simulink model "algorithm"  (R2026a)
settings: Solver=FixedStepDiscrete  FixedStep=foc.Ts
PreLoadFcn:
  | if exist('init', 'file') ~= 2,   pDir = fileparts(fileparts(which(bdroot)));   if isempty(pDir), pDir = pwd; end;   addpath(fullfile(pDir, 'scripts'));   addpath(fullfile(pDir, 'models'));   addpath(pDir); end; init;
InitFcn:
  | if exist('init', 'file') ~= 2,   pDir = fileparts(fileparts(which(bdroot)));   if isempty(pDir), pDir = pwd; end;   addpath(fullfile(pDir, 'scripts'));   addpath(fullfile(pDir, 'models'));   addpath(pDir); end; init;
undefined symbols (not defined in the file): calibration_modulation, calibration_request, control_enable_request, control_fault_reset, control_mode_request, current_offset_counts, DiscIntNeverNeededParam, foc, has_stored_resolver_offset, open_loop_electrical_hz, open_loop_modulation, pmsm, resolver_angle_offset, sensor, torque_ref_nm
libraries: mcbeeMathTransformLib x3, slpidlib x3, mcbcontrolslib x3, simulink x2, mcbpositiondecoderlib x1
(part 2 of 2)

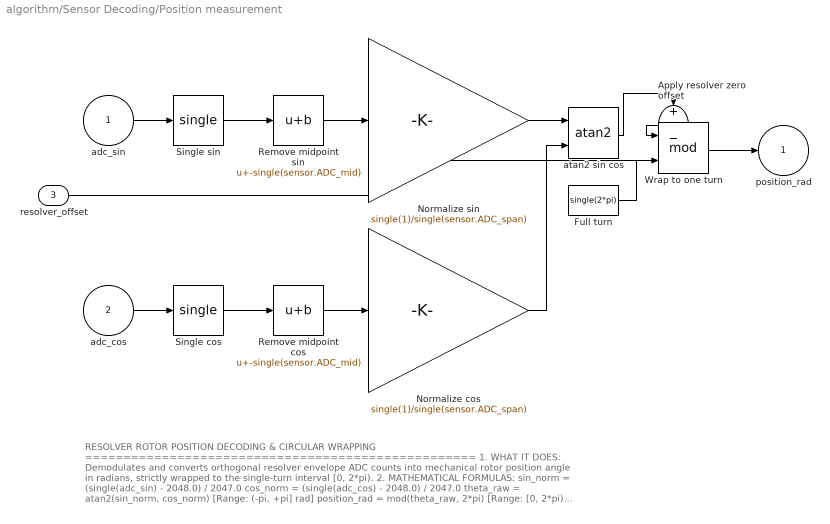
== system algorithm/Sensor Decoding/Position measurement ==
  note: RESOLVER ROTOR POSITION DECODING & CIRCULAR WRAPPING
      | ===================================================
      | 1. WHAT IT DOES:
      | Demodulates and converts orthogonal resolver envelope ADC counts into mechanical rotor
      | position angle in radians, strictly wrapped to the single-turn interval [0, 2*pi).
      |
      | 2. MATHEMATICAL FORMULAS:
      |   sin_norm = (single(adc_sin) - 2048.0) / 2047.0
      |   cos_norm = (single(adc_cos) - 2048.0) / 2047.0
      |   theta_raw = atan2(sin_norm, cos_norm)           [Range: (-pi, +pi] rad]
      |   position_rad = mod(theta_raw, 2*pi)             [Range: [0, 2*pi) rad]
      |
      | 3. WHY IT IS NEEDED:
      | Field-Oriented Control requires accurate, continuous knowledge of rotor position to align
      | the Park and Clarke reference frames. Using atan2(sin, cos) provides amplitude-invariant
      | angle reconstruction that rejects common-mode excitation variations and noise. Wrapping to
      | [0, 2*pi) provides a clean, standardized mechanical coordinate system for electrical angle derivation.
  adc_sin : Inport  OutDataTypeStr=uint16
  adc_cos : Inport  Port=2  OutDataTypeStr=uint16
  resolver_offset : Inport  Port=3
  Apply resolver zero offset : Sum  Inputs=+-
  Full turn : Constant  Value=single(2*pi)
  Normalize cos : Gain  Gain=single(1)/single(sensor.ADC_span)
  Normalize sin : Gain  Gain=single(1)/single(sensor.ADC_span)
  Remove midpoint cos : Bias  Bias=-single(sensor.ADC_mid)
  Remove midpoint sin : Bias  Bias=-single(sensor.ADC_mid)
  Single cos : DataTypeConversion  OutDataTypeStr=single
  Single sin : DataTypeConversion  OutDataTypeStr=single
  Wrap to one turn : Math  Operator=mod
  atan2 sin cos : Trigonometry  Operator=atan2
  position_rad : Outport
  wires:
  Wrap to one turn/1 -> position_rad/1
  Normalize cos/1 -> atan2 sin cos/2
  Normalize sin/1 -> atan2 sin cos/1
  Remove midpoint cos/1 -> Normalize cos/1
  adc_cos/1 -> Single cos/1
  Remove midpoint sin/1 -> Normalize sin/1
  Single cos/1 -> Remove midpoint cos/1
  Single sin/1 -> Remove midpoint sin/1
  Full turn/1 -> Wrap to one turn/2
  adc_sin/1 -> Single sin/1
  atan2 sin cos/1 -> Apply resolver zero offset/1
  Apply resolver zero offset/1 -> Wrap to one turn/1
  resolver_offset/1 -> Apply resolver zero offset/2

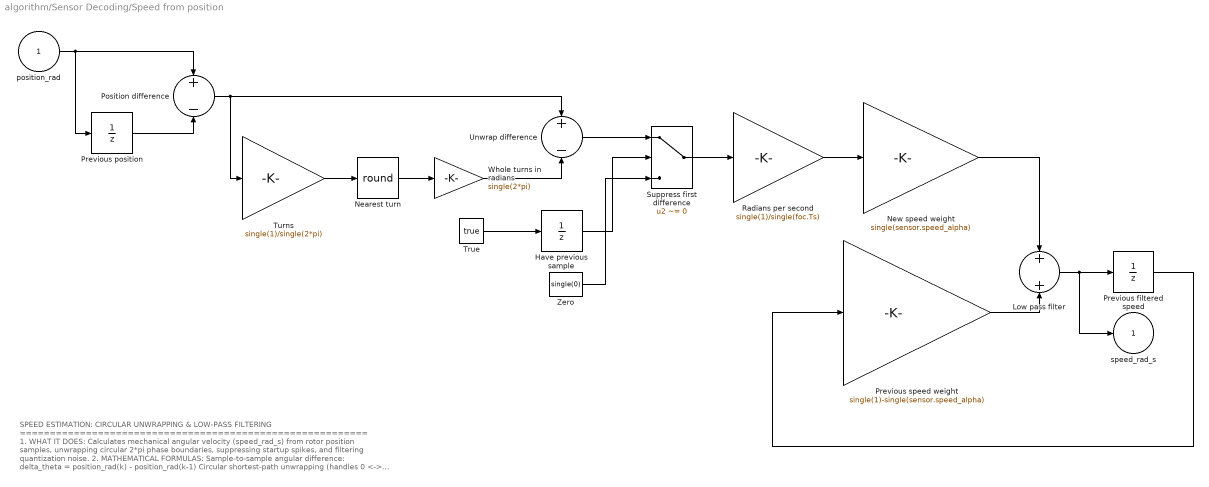
== system algorithm/Sensor Decoding/Speed from position ==
  note: SPEED ESTIMATION: CIRCULAR UNWRAPPING & LOW-PASS FILTERING
      | ==========================================================
      | 1. WHAT IT DOES:
      | Calculates mechanical angular velocity (speed_rad_s) from rotor position samples,
      | unwrapping circular 2*pi phase boundaries, suppressing startup spikes, and filtering
      | quantization noise.
      |
      | 2. MATHEMATICAL FORMULAS:
      | Sample-to-sample angular difference:
      |   delta_theta = position_rad(k) - position_rad(k-1)
      |
      | Circular shortest-path unwrapping (handles 0 <-> 2*pi transitions):
      |   delta_theta_unwrap = delta_theta - 2*pi * round(delta_theta / (2*pi))
      |
      | Differentiated raw speed (with first-step startup suppression):
      |   omega_raw(1) = 0
      |   omega_raw(k) = delta_theta_unwrap / Ts          [Ts = 50 us (20 kHz)]
      |
      | Discrete 1st-order Low-Pass Filter (cutoff fc = 150 Hz):
      |   omega_filt(k) = (1 - alpha) * omega_filt(k-1) + alpha * omega_raw(k)
      |   alpha = (2*pi * fc * Ts) / (1 + 2*pi * fc * Ts) ≈ 0.04505
      |
      | 3. WHY IT IS NEEDED:
      | - Boundary Wrap Immunity: As the rotor rotates past 2*pi -> 0 or 0 -> 2*pi, delta_theta
      |   would jump by +/-2*pi, producing an enormous false velocity spike (+/-125,663 rad/s).
      |   Shortest-path unwrapping eliminates this completely.
      | - Startup Quiescence: Suppressing the first step prevents false speed kicks when starting
      |   from a nonzero stationary angle.
      | - Noise Rejection: Differentiating quantized 12-bit ADC resolver signals amplifies high-
      |   frequency quantization noise; the 150 Hz LPF smooths the velocity signal for stable speed
      |   and current loop feedback.
  position_rad : Inport  OutDataTypeStr=single
  Have previous sample : UnitDelay  InitialCondition=false  SampleTime=foc.Ts
  Low pass filter : Sum
  Nearest turn : Rounding  Operator=round
  New speed weight : Gain  Gain=single(sensor.speed_alpha)
  Position difference : Sum  Inputs=+-
  Previous filtered speed : UnitDelay  InitialCondition=single(0)  SampleTime=foc.Ts
  Previous position : UnitDelay  InitialCondition=single(0)  SampleTime=foc.Ts
  Previous speed weight : Gain  Gain=single(1)-single(sensor.speed_alpha)
  Radians per second : Gain  Gain=single(1)/single(foc.Ts)
  Suppress first difference : Switch  Criteria=u2 ~= 0
  True : Constant  Value=true
  Turns : Gain  Gain=single(1)/single(2*pi)
  Unwrap difference : Sum  Inputs=+-
  Whole turns in radians : Gain  Gain=single(2*pi)
  Zero : Constant  Value=single(0)
  speed_rad_s : Outport
  wires:
  Previous filtered speed/1 -> Previous speed weight/1
  Previous speed weight/1 -> Low pass filter/2
  New speed weight/1 -> Low pass filter/1
  Radians per second/1 -> New speed weight/1
  Unwrap difference/1 -> Suppress first difference/1
  Position difference/1 -> Turns/1, Unwrap difference/1
  Nearest turn/1 -> Whole turns in radians/1
  Suppress first difference/1 -> Radians per second/1
  position_rad/1 -> Previous position/1, Position difference/1
  Turns/1 -> Nearest turn/1
  Low pass filter/1 -> speed_rad_s/1, Previous filtered speed/1
  Have previous sample/1 -> Suppress first difference/2
  Zero/1 -> Suppress first difference/3
  Whole turns in radians/1 -> Unwrap difference/2
  Previous position/1 -> Position difference/2
  True/1 -> Have previous sample/1

== matlab function algorithm/Sensor Offset Calibration/Average and store offsets ==
  data: ia input size=1; current_offsets output size=[3]; ib input size=1; ic input size=1; rsin input size=1; rcos input size=1; current_enable input size=1; resolver_enable input size=1; current_initial input size=[3]; resolver_initial input size=1; resolver_offset output size=1; current_done output size=1; resolver_done output size=1
function [current_offsets, resolver_offset, current_done, resolver_done] = calibrate(ia, ib, ic, rsin, rcos, current_enable, resolver_enable, current_initial, resolver_initial)
%#codegen
% Signal averaging belongs in Simulink. Stateflow only enables each phase.
persistent current_store resolver_store current_sum resolver_sin_sum resolver_cos_sum current_count resolver_count previous_current_enable previous_resolver_enable
if isempty(current_store)
    current_store = single(current_initial);
    resolver_store = single(resolver_initial);
    current_sum = single([0;0;0]);
    resolver_sin_sum = single(0); resolver_cos_sum = single(0);
    current_count = uint32(0); resolver_count = uint32(0);
    previous_current_enable = false; previous_resolver_enable = false;
end
current_done = false; resolver_done = false;
if current_enable
    if ~previous_current_enable
        current_sum = single([0;0;0]); current_count = uint32(0);
    end
    if current_count < uint32(10000)
        current_sum = current_sum + single([ia;ib;ic]);
        current_count = current_count + uint32(1);
    end
    if current_count >= uint32(10000)
        current_store = current_sum / single(current_count); current_done = true;
    end
end
if resolver_enable
    if ~previous_resolver_enable
        resolver_sin_sum = single(0); resolver_cos_sum = single(0); resolver_count = uint32(0);
    end
    if resolver_count < uint32(10000)
        resolver_sin_sum = resolver_sin_sum + single(rsin) - single(2048);
        resolver_cos_sum = resolver_cos_sum + single(rcos) - single(2048);
        resolver_count = resolver_count + uint32(1);
    end
    if resolver_count >= uint32(10000)
        resolver_store = atan2(resolver_sin_sum, resolver_cos_sum); resolver_done = true;
    end
end
previous_current_enable = current_enable;
previous_resolver_enable = resolver_enable;
current_offsets = current_store;
resolver_offset = resolver_store;
end

== matlab function algorithm/Protection Monitor ==
  data: currents input single size=[3]; fault output boolean size=1; speed input single size=1; ia input uint16 size=1; ib input uint16 size=1; ic input uint16 size=1; rsin input uint16 size=1; rcos input uint16 size=1; reset input; fault_flags output
function [fault, fault_flags] = protection_monitor(currents, speed, ia, ib, ic, rsin, rcos, reset)
%#codegen
rawCurrent = abs(single(currents));
oc_u = rawCurrent(1) > single(0.90);
oc_v = rawCurrent(2) > single(0.90);
oc_w = rawCurrent(3) > single(0.90);
overcurrent = oc_u || oc_v || oc_w;

overspeed = abs(speed) > single(2094.3951);

rail_low  = (ia <= uint16(8)) || (ib <= uint16(8)) || (ic <= uint16(8));
rail_high = (ia >= uint16(4087)) || (ib >= uint16(4087)) || (ic >= uint16(4087));
adcRail   = rail_low || rail_high;

s = (single(rsin) - single(2048)) / single(2047);
c = (single(rcos) - single(2048)) / single(2047);
amp = sqrt(s*s + c*c);
res_low  = amp < single(0.10);
res_high = amp > single(1.30);
resolverBad = res_low || res_high;

persistent bad_count latched_flags
if isempty(bad_count)
    bad_count = uint16(0);
    latched_flags = uint32(0);
end

bad = overcurrent || overspeed || adcRail || resolverBad;
if bad
    if bad_count < uint16(100)
        bad_count = bad_count + uint16(1);
    end
else
    bad_count = uint16(0);
end

fault = (bad_count >= uint16(100));

% Active fault bits:
active_flags = uint32(0);
if oc_u,      active_flags = bitor(active_flags, uint32(1)); end    % Bit 0: Overcurrent U
if oc_v,      active_flags = bitor(active_flags, uint32(2)); end    % Bit 1: Overcurrent V
if oc_w,      active_flags = bitor(active_flags, uint32(4)); end    % Bit 2: Overcurrent W
if overspeed, active_flags = bitor(active_flags, uint32(8)); end    % Bit 3: Overspeed
if rail_low,  active_flags = bitor(active_flags, uint32(16)); end   % Bit 4: ADC Rail Low
if rail_high, active_flags = bitor(active_flags, uint32(32)); end   % Bit 5: ADC Rail High
if res_low,   active_flags = bitor(active_flags, uint32(64)); end   % Bit 6: Resolver Amp Low
if res_high,  active_flags = bitor(active_flags, uint32(128)); end  % Bit 7: Resolver Amp High
if fault,     active_flags = bitor(active_flags, uint32(256)); end  % Bit 8: Trip Latched

if reset
    latched_flags = active_flags;
else
    latched_flags = bitor(latched_flags, active_flags);
end

fault_flags = latched_flags;
end

== stateflow chart algorithm/Operating Mode Supervisor ==
  state IDLE
    entry:
    supervisor_state = SupervisorState.IDLE;
    active_mode = uint8(0);
    pwm_enable = false;
    current_cal_enable = false;
    resolver_align_enable = false;
    resolver_sample_enable = false;
    fault_latched = false;
    during:
    if calibration_request == uint8(0)
    cal_request_processed = false;
    end
  state READY
    entry:
    supervisor_state = SupervisorState.READY;
    active_mode = uint8(0);
    pwm_enable = false;
    current_cal_enable = false;
    resolver_align_enable = false;
    resolver_sample_enable = false;
    fault_latched = false;
    during:
    if ~enable_request
    reenable_required = false;
    end
    if calibration_request == uint8(0)
    cal_request_processed = false;
    end
  state RUN
    entry:
    supervisor_state = SupervisorState.RUN;
    run_mode = mode_request;
    active_mode = run_mode;
    pwm_enable = true;
    current_cal_enable = false;
    resolver_align_enable = false;
    resolver_sample_enable = false;
    fault_latched = false;
    during:
    active_mode = run_mode;
    if calibration_request == uint8(0)
    cal_request_processed = false;
    end
  state CALIBRATION
    entry:
    supervisor_state = SupervisorState.CALIBRATION;
    active_mode = uint8(0);
    pwm_enable = false;
    current_cal_enable = false;
    resolver_align_enable = false;
    resolver_sample_enable = false;
    do_current_cal = ~startup_current_cal_done || calibration_request == uint8(1) || calibration_request == uint8(3);
    do_angle_cal = ~has_stored_angle || calibration_request == uint8(2) || calibration_request == uint8(3);
    fault_latched = false;
    state CURRENT_CAL
      entry:
      current_cal_enable = true;
      pwm_enable = false;
      resolver_align_enable = false;
      resolver_sample_enable = false;
      exit:
      current_cal_enable = false;
      startup_current_cal_done = true;
    state ANGLE_ALIGN
      entry:
      current_cal_enable = false;
      pwm_enable = true;
      resolver_align_enable = true;
      resolver_sample_enable = false;
      ticks = uint32(0);
      during:
      ticks = ticks + uint32(1);
    state ANGLE_SAMPLE
      entry:
      current_cal_enable = false;
      pwm_enable = true;
      resolver_align_enable = true;
      resolver_sample_enable = true;
    state CAL_DONE
      entry:
      current_cal_enable = false;
      pwm_enable = false;
      resolver_align_enable = false;
      resolver_sample_enable = false;
      cal_request_processed = true;
    state SELECT_CALIBRATION
      entry:
      pwm_enable = false;
    CURRENT_CAL -> ANGLE_ALIGN [order 1] : [current_cal_done && do_angle_cal]
    ANGLE_ALIGN -> ANGLE_SAMPLE : [ticks >= uint32(20000)]
    ANGLE_SAMPLE -> CAL_DONE : [resolver_cal_done]
    SELECT_CALIBRATION -> CURRENT_CAL [order 1] : [do_current_cal]
    CURRENT_CAL -> CAL_DONE [order 2] : [current_cal_done && ~do_angle_cal]
    SELECT_CALIBRATION -> ANGLE_ALIGN [order 2] : [~do_current_cal && do_angle_cal]
    SELECT_CALIBRATION -> CAL_DONE [order 3]
  state FAULT
    entry:
    supervisor_state = SupervisorState.FAULT;
    active_mode = uint8(0);
    pwm_enable = false;
    current_cal_enable = false;
    resolver_align_enable = false;
    resolver_sample_enable = false;
    fault_latched = true;
  RUN -> IDLE [order 2] : [mode_request == uint8(0) || mode_request > uint8(3)]
  (default) -> SELECT_CALIBRATION [order 1]
  (default) -> IDLE [order 2]
  IDLE -> CALIBRATION [order 1] : [~startup_current_cal_done || (calibration_request ~= uint8(0) && ~cal_request_processed)]
  IDLE -> FAULT [order 3] : [fault_active]
  RUN -> FAULT [order 3] : [fault_active]
  IDLE -> READY [order 2] : [startup_current_cal_done && mode_request >= uint8(1) && mode_request <= uint8(3)]
  READY -> IDLE [order 2] : [mode_request == uint8(0)]
  READY -> RUN [order 1] : [enable_request && ~reenable_required && mode_request >= uint8(1) && mode_request <= uint8(3)]
  RUN -> READY [order 1] : [~enable_request || mode_request ~= run_mode]{reenable_required = enable_request;}
  CALIBRATION -> IDLE [order 2] : [cal_request_processed && mode_request == uint8(0)]
  FAULT -> IDLE : [reset_fault && ~fault_active]
  READY -> CALIBRATION [order 3] : [calibration_request ~= uint8(0) && ~cal_request_processed]
  CALIBRATION -> READY [order 1] : [cal_request_processed && mode_request ~= uint8(0)]
  READY -> FAULT [order 4] : [fault_active]
  CALIBRATION -> FAULT [order 3] : [fault_active]
  data: mode_request input uint8 size=1; enable_request input boolean size=1; calibration_request input uint8 size=1; fault_active input boolean size=1; reset_fault input boolean size=1; current_cal_done input boolean size=1; resolver_cal_done input boolean size=1; has_stored_angle input boolean size=1; active_mode output uint8 size=1; pwm_enable output boolean size=1; current_cal_enable output boolean size=1; resolver_align_enable output boolean size=1; resolver_sample_enable output boolean size=1; fault_latched output boolean size=1; supervisor_state output Enum: SupervisorState size=1; startup_current_cal_done local boolean size=1 =false; cal_request_processed local boolean size=1 =false; ticks local uint32 size=1 =0; do_current_cal local boolean size=1 =false; do_angle_cal local boolean size=1 =false; run_mode local uint8 size=1 =0; reenable_required local boolean size=1 =false
